simulink model "Comment_Uncomment"  (R2020a)
settings: Solver=VariableStepAuto  StartTime=0.0  StopTime=10.0  RelTol=1e-3
settings Model: Creator=royde  LastModifiedBy=royde

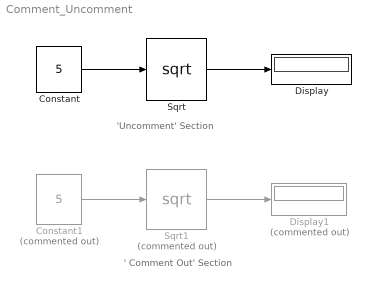
== system Comment_Uncomment ==
  note: ' Comment Out' Section
  note: 'Uncomment' Section
  Constant : Constant  Value=5
  Constant1 : Constant  Commented=on  Value=5
  Display : Display
  Display1 : Display  Commented=on
  Sqrt : Sqrt  SaturateOnIntegerOverflow=on
  Sqrt1 : Sqrt  Commented=on  SaturateOnIntegerOverflow=on
  wires:
  Constant1/1 -> Sqrt1/1
  Constant/1 -> Sqrt/1
  Sqrt/1 -> Display/1
  Sqrt1/1 -> Display1/1
